simulink model "CSAD_PIDcontroller_ny"  (R2016b)
settings: Solver=ode3  StartTime=0.0  StopTime=tend  FixedStep=0.01  RelTol=1e-3  EnableMultiTasking=on
undefined symbols (not defined in the file): C, Cdn, Cdt, Cmn, d, D, depCur, des_pos, E, emfact, eps_c, epsilon, hd, hd2, Hoerner, I_s, k_cc, K_d_psi, K_d_x, K_d_y, K_i_psi, K_i_x, K_i_y, K_omega, K_p_psi, K_p_x, K_p_y, Kp, Kq, Kqr, Kt, Ktr, L, Max_Acceleration, Max_rotation, Max_thrust, moorLineProp, n_c, n_max, p_cc, P_max, Q_f0, Q_max, r0, r_cc, r_dot0, rBottomEnd, Rho, rhoCab, rhoWat, stiffSeafloor, T_psi, T_x, T_y, Thruster, Thruster_control, Thruster_lock, velCur, vessel, vesselABC ... (+7)
libraries: marine_gnc x9, dspmtrx3 x6, simulink x6, simulink_extras x3, marine_hydro x3
(part 3 of 5)

== matlab function CSAD_PIDcontroller_ny/Virtual CS Inocean Cat I Drillship 6 DOF/FEM mooring/Mooring Line 2/FEM mooring cable ==
  data: state input; rBottomEnd input; rTopEnd input; state_dot output; E input; d input; L input; rhoCab input; rhoWat input; emfact input; stiffSeafloor input; Cmn input; Cdt input; Cdn input; depCur input; velCur input; Ftop output; waterDepth input
function [state_dot, Ftop]  = fcn(state,rBottomEnd,rTopEnd,E,d,L,rhoCab,rhoWat,emfact,stiffSeafloor,Cmn,Cdt,Cdn,depCur,velCur,waterDepth)
% This is a sophisticated FEM model which is used to describe the cable. It
% contain the following parameters.
%   Coordinate
%       local NED reference: calm water sea surface z=0, positive upward

%   Outputs:
%       r_ddot	---     acceleration of each nodes
%       Ftop	---     top end restoring force
%       Fbottom ---     bottom end restoring force

%   Input variables:
%       r       ---     positions of nodes [3*(numNode-1),1]
%       r_dot   ---     velocities of nodes [3*(numNode-1),1]
%       rBottomEnd	--- bottom point       [3,1]
%       topEnd      --- top point       [3,1]

%   Initial conditions:
%       r0      ---     initial positionsof nodes   [3*(numNode),1]
%       r_dot0  ---     initial velocities of nodes [3*(numNode),1]

%   Constant parameters:
%       E       ---     elastic modulus
%       d       ---     diameter of the cable
%       A0      ---     area of the cable (A0=pi/4*d^2)
%       L       ---     length of the cable
%       numNode	---     number of the nodes (excluded the anchor)        
%       rhoCab	---     cable density
%       rhoWat	---     water density
%       ef      ---     factor for stiffness calculation in the reaction force,[1,1], e.g. ef=1;
%       Cmn     ---     added mass coefficient in mass matrix, [1,1]
%       Cdt     ---     tangential drag coefficient in drag force, [1,1]
%       Cdn     ---     normal drag coefficient in drag force, [1,1]
%       depCur  ---     current depth vector (botom to water surface)  [numCur,1]
%       velCur  ---     current velocity vector             [3*numCur,1]
%       deltaT  ---     time difference between two process, [1,1]

%   Other parameters in the program:
%       l       ---     length of each segment, [numNode-1,1]  
%       l_k   --- 	[3*(numNode-1),1]           Eq.9
%       epsilon_k   ---     strain, [numNode-1,1]     Eq.9
%       rho0    ---     mass per unit length of unstrethched cable, [1,1]
%       vc      ---     velicity of current at each node, [3*(numCur+1),1]
%       numCur  ---     number of point in the current profile
%       numNodeSeaFloor     --- number of node on the sea floor
%       f_k_r   ---     reaction force at each node, [3*(numCur+1),1]               Eq.17
%       f_k_hg  ---     hydrostatic force & gravity at each node, [3*(numCur+1),1]  Eq.17
%       f_k_d   ---     drag force at each node, [3*(numCur+1),1]                   Eq.17
%       P_k     ---     (l_k*l_k')/epsilon_k^2                                      Eq.19
%       m_k     ---     mass matrix of each node, [3,3]
%       r_ddot  ---     acceleration of nodes [3*(numNode+1),1]                     Eq.17


%   Note that :
	 % i=k in {l_k,epsilon_k,vc,f_k_r,f_k_hg,f_k_g,r,r_dot,m_k} [k=1,...,n-1],
            
%   Reference:
%       Aamo, O. M. and T. I. Fossen (2001). "Finite Element Modelling of 
%       Moored Vessels." Mathematical and Computer Modelling of Dynamical 
%       Systems 7(1): 47-75.

% Author: Zhengru Ren, NTNU
%% Constants statement
numNode     =   20;
% persistent numNode
% if isempty(numNode)
% numNode=numNode1;
% end

l   =   L/numNode*ones(1,numNode);      % length per segment (m)
g   =   9.81;                           % gravity acceleration (m/s^2)
A0  =   pi/4*d^2;                       % area (m^2)
rho0=   rhoCab*A0; 
C1  =   Cmn*A0*rhoWat;
C2  =   0.5*Cdt*d*rhoWat;
C3  =   0.5*Cdn*d*rhoWat;

r   =   state(1:3*numNode-3);
r_dot   =   state(3*numNode-2:6*numNode-6);

%% Current velocity resample for each node
vc      =   zeros(3*(numNode-1),1);
for i = 1 : numNode-1
    if r(3*i)  >  waterDepth
        vc(3*i-2:3*i)   =  [0;0;0]; % below or on the seafloor
    elseif r(3*i)  >=  depCur(end) % below the bottom current point (below the seabed)
        vc(3*i-2:3*i)   =  velCur(end-2:end);
    elseif  r(3*i)  <=  depCur(1) % above the top current point (above water surface)
        vc(3*i-2:3*i)   =   velCur(1:3);
    else
        cur=max(find(depCur<=r(3*i)));       
        vc(3*i-2:3*i)   =   velCur(3*cur-2:3*cur)+...
            (velCur(3*cur+1:3*cur+3)-velCur(3*cur-2:3*cur))./...
            (depCur(cur+1)-depCur(cur)).*(r(3*i)-depCur(cur));
    end
end
% r(3:3:end)
% vc
%% Basic parameter update
l_k         =   zeros(3*numNode,1);
epsilon_k   =   zeros(numNode,1);

l_k(1:3,1)	=	r(1:3,1)-rBottomEnd;
epsilon_k(1,1)      =   norm(l_k(1:3,1),2);
for i = 2 : numNode-1
    l_k(3*i-2:3*i,1)    =   r(3*i-2:3*i,1)-r(3*(i-1)-2:3*(i-1),1); % [NOTE]
    epsilon_k(i,1)      =   norm(l_k(3*i-2:3*i,1),2);
end
l_k(3*numNode-2:3*numNode,1)	=	rTopEnd-r(3*(numNode-1)-2:3*(numNode-1),1);
epsilon_k(numNode,1)      =   norm(l_k(3*numNode-2:3*numNode,1),2);


%% External forces
% Reaction force
f_k_r       =   zeros(3*(numNode),1);
f_k_hg      =   zeros(3*(numNode),1);
f_k_d       =   zeros(3*(numNode),1);
f_tol       =   zeros(3*(numNode),1);
r_ddot  =   zeros(3*(numNode-1),1);

f_k_hg(3)	=	f_k_hg(3)+0.5*l(1)*A0*(rhoCab-rhoWat)*g;
f_k_r(1:3)	=   f_k_r(1:3)-E*A0*emfact*((1/l(1)-1/epsilon_k(1))*l_k(1:3));
for i = 1:numNode-1
    f_k_r(3*i-2:3*i)	=   f_k_r(3*i-2:3*i)+E*A0*emfact*((1/l(i+1)-1/epsilon_k(i+1))*l_k(3*i+1:3*i+3));
    f_k_r(3*i+1:3*i+3)	=   f_k_r(3*i+1:3*i+3)-E*A0*emfact*((1/l(i+1)-1/epsilon_k(i+1))*l_k(3*i+1:3*i+3));
    %     E*A0*emfact*((1/l(i)-1/epsilon_k(i))*l_k(3*i-2:3*i) - (1/l(i+1)-1/epsilon_k(i+1))*l_k(3*i+1:3*i+3));
    

    % Hydrostatic force & gravity
    if r(3*i) < waterDepth-2  % above the seafloor(-2 safety value)
        f_k_hg(3*i)	=	f_k_hg(3*i)+0.5*l(i+1)*A0*(rhoCab-rhoWat)*g;
        f_k_hg(3*i+3)	=	f_k_hg(3*i+3)+0.5*l(i+1)*A0*(rhoCab-rhoWat)*g;
    else % below or on the seafloor
        f_k_hg(3*i)	=   stiffSeafloor*(waterDepth-r(3*i));
    end

    % Drag force
    P_k         =   l_k(3*i-2:3*i)*l_k(3*i-2:3*i)'./(epsilon_k(i)^2);
    P_kplus1    =   l_k(3*i+1:3*i+3)*l_k(3*i+1:3*i+3)'./(epsilon_k(i+1)^2); 
    f_k_d(3*i-2:3*i)	=   -0.5*(  C2*(...
                                abs((r_dot(3*i-2:3*i)-vc(3*i-2:3*i))'*l_k(3*i-2:3*i))*P_k+...
                                abs((r_dot(3*i-2:3*i)-vc(3*i-2:3*i))'*l_k(3*i+1:3*i+3))*P_kplus1...
                                        )...   % dt
                                 +  C3*(...
                                epsilon_k(i)*norm((eye(3)-P_k)*(r_dot(3*i-2:3*i)-vc(3*i-2:3*i)))*(eye(3)-P_k)+...
                                epsilon_k(i+1)*norm((eye(3)-P_kplus1)*(r_dot(3*i-2:3*i)-vc(3*i-2:3*i)))*(eye(3)-P_kplus1)...
                                        )...    % dn
                                )*(r_dot(3*i-2:3*i)-vc(3*i-2:3*i));
                            
    f_tol(3*i-2:3*i)   =   f_k_hg(3*i-2:3*i)+f_k_d(3*i-2:3*i)+f_k_r(3*i-2:3*i); 	% total force
                        
	m_k     =   (rho0*l(i)+0.5*C1*(epsilon_k(i)+epsilon_k(i+1)))*eye(3)-0.5*C1*(l_k(3*i-2:3*i)*l_k(3*i-2:3*i)'/epsilon_k(i)+l_k(3*i+1:3*i+3)*l_k(3*i+1:3*i+3)'/epsilon_k(i+1));
	AAA=(m_k(3,3)*m_k(1,2)^2 - 2*m_k(1,2)*m_k(1,3)*m_k(2,3) + m_k(2,2)*m_k(1,3)^2 + m_k(1,1)*m_k(2,3)^2 - m_k(1,1)*m_k(2,2)*m_k(3,3));
    r_ddot(3*i-2:3*i,1)	=   [ -(- m_k(2,3)^2 + m_k(2,2)*m_k(3,3))/AAA,    (m_k(1,2)*m_k(3,3) - m_k(1,3)*m_k(2,3))/AAA,   -(m_k(1,2)*m_k(2,3) - m_k(1,3)*m_k(2,2))/AAA;
        (m_k(1,2)*m_k(3,3) - m_k(1,3)*m_k(2,3))/AAA, -(- m_k(1,3)^2 + m_k(1,1)*m_k(3,3))/AAA,   -(m_k(1,2)*m_k(1,3) - m_k(1,1)*m_k(2,3))/AAA;
        -(m_k(1,2)*m_k(2,3) - m_k(1,3)*m_k(2,2))/AAA,   -(m_k(1,2)*m_k(1,3) - m_k(1,1)*m_k(2,3))/AAA, -(- m_k(1,2)^2 + m_k(1,1)*m_k(2,2))/AAA]*f_tol(3*i-2:3*i);
end


%% Mass matrix & acceleration
% for i = 1:numNode-1
%     m_k     =   (rho0*l(i)+0.5*C1*(epsilon_k(i)+epsilon_k(i+1)))*eye(3)-0.5*C1*(l_k(3*i-2:3*i)*l_k(3*i-2:3*i)'/epsilon_k(i)+l_k(3*i+1:3*i+3)*l_k(3*i+1:3*i+3)'/epsilon_k(i+1));
% %   (1)     r_ddot(3*i-2:3*i,1)	=	m_k\f_tol(3*i-2:3*i);
% %   (2)     
% AAA=(m_k(3,3)*m_k(1,2)^2 - 2*m_k(1,2)*m_k(1,3)*m_k(2,3) + m_k(2,2)*m_k(1,3)^2 + m_k(1,1)*m_k(2,3)^2 - m_k(1,1)*m_k(2,2)*m_k(3,3));
% r_ddot(3*i-2:3*i,1)	=   [ -(- m_k(2,3)^2 + m_k(2,2)*m_k(3,3))/AAA,    (m_k(1,2)*m_k(3,3) - m_k(1,3)*m_k(2,3))/AAA,   -(m_k(1,2)*m_k(2,3) - m_k(1,3)*m_k(2,2))/AAA;
%     (m_k(1,2)*m_k(3,3) - m_k(1,3)*m_k(2,3))/AAA, -(- m_k(1,3)^2 + m_k(1,1)*m_k(3,3))/AAA,   -(m_k(1,2)*m_k(1,3) - m_k(1,1)*m_k(2,3))/AAA;
%     -(m_k(1,2)*m_k(2,3) - m_k(1,3)*m_k(2,2))/AAA,   -(m_k(1,2)*m_k(1,3) - m_k(1,1)*m_k(2,3))/AAA, -(- m_k(1,2)^2 + m_k(1,1)*m_k(2,2))/AAA]*f_tol(3*i-2:3*i);
% 
% %   (3)
% % m1=[m_k(1,1),m_k(1,2),m_k(1,3),m_k(2,2),m_k(2,3),m_k(3,3)];F=f_tol(3*i-2:3*i);
% % a12=m_k(1,2);a13=m_k(1,3);a23=m_k(2,3);
% % m1(2)=m1(2)/m1(1);
% % m1(3)=m1(3)/m1(1);
% % F(1)=F(1)/m1(1);
% % m1(5)=(m1(5)-a12*m1(3))/(m1(4)-a12*m1(2));
% % F(2)=(F(2)-a12*F(1))/(m1(4)-a12*m1(2));		
% % m1(6)=m1(6)-a13*m1(3)-m1(5)*(a23-a13*m1(2));
% % r_ddot(3*i,1)=(F(3)-a13*F(1)-F(2)*(a23-a13*m1(2)))/m1(6);
% % r_ddot(3*i-1,1)=F(2)-m1(5)*F(3);
% % r_ddot(3*i-2,1)=F(1)-m1(2)*F(2)+m1(3)*F(3);    
% end

state_dot = [r_dot;r_ddot];

%% Seafloor resample for each node (if the seafloor is not flat)
% numNodeSeaFloor     =
% xNodeSeaFloor	=   zeros(numNodeSeaFloor,1);
% yNodeSeaFloor	=   zeros(numNodeSeaFloor,1);
% zNodeSeaFloorZ	=   zeros(numNodeSeaFloor,1);
% 
% for i=1:numNodeSeaFloor
%     xNodeSeaFloor(i,1)	=	r(3*i-2,1);
%     yNodeSeaFloor(i,1)	=   r(3*i-2,1);
% end
% zNodeSeaFloorZ  =   interp2(seaFloor(:,1),seaFloor(:,2),seaFloor(:,3),xNodeSeaFloor,yNodeSeaFloor);
% zNodeSeaFloorZ   =   waterDepth*ones(numNode+1,1);

%% Restoring forces at the top end and bottom end
% Bottom end
% Fbottom         =   E*A0*emfact*(1/l(1)-1/epsilon_k(1)) * l_k(1:3);

% Top end
Ftop            =   -E*A0*emfact*(1/l(numNode)-1/epsilon_k(numNode)) * l_k(3*numNode-2:3*numNode);

== matlab function CSAD_PIDcontroller_ny/Virtual CS Inocean Cat I Drillship 6 DOF/FEM mooring/Mooring Line 1/FEM mooring cable ==
  data: state input; rBottomEnd input; rTopEnd input; state_dot output; E input; d input; L input; rhoCab input; rhoWat input; emfact input; stiffSeafloor input; Cmn input; Cdt input; Cdn input; depCur input; velCur input; Ftop output; waterDepth input
function [state_dot, Ftop]  = fcn(state,rBottomEnd,rTopEnd,E,d,L,rhoCab,rhoWat,emfact,stiffSeafloor,Cmn,Cdt,Cdn,depCur,velCur,waterDepth)
% This is a sophisticated FEM model which is used to describe the cable. It
% contain the following parameters.
%   Coordinate
%       local NED reference: calm water sea surface z=0, positive upward

%   Outputs:
%       r_ddot	---     acceleration of each nodes
%       Ftop	---     top end restoring force
%       Fbottom ---     bottom end restoring force

%   Input variables:
%       r       ---     positions of nodes [3*(numNode-1),1]
%       r_dot   ---     velocities of nodes [3*(numNode-1),1]
%       rBottomEnd	--- bottom point       [3,1]
%       rtopEnd      --- top point       [3,1]

%   Initial conditions:
%       r0      ---     initial positionsof nodes   [3*(numNode),1]
%       r_dot0  ---     initial velocities of nodes [3*(numNode),1]

%   Constant parameters:
%       E       ---     elastic modulus
%       d       ---     diameter of the cable
%       A0      ---     area of the cable (A0=pi/4*d^2)
%       L       ---     length of the cable
%       numNode	---     number of the nodes (excluded the anchor)        
%       rhoCab	---     cable density
%       rhoWat	---     water density
%       ef      ---     factor for stiffness calculation in the reaction force,[1,1], e.g. ef=1;
%       Cmn     ---     added mass coefficient in mass matrix, [1,1]
%       Cdt     ---     tangential drag coefficient in drag force, [1,1]
%       Cdn     ---     normal drag coefficient in drag force, [1,1]
%       depCur  ---     current depth vector (botom to water surface)  [numCur,1]
%       velCur  ---     current velocity vector             [3*numCur,1]
%       deltaT  ---     time difference between two process, [1,1]

%   Other parameters in the program:
%       l       ---     length of each segment, [numNode-1,1]  
%       l_k   --- 	[3*(numNode-1),1]           Eq.9
%       epsilon_k   ---     strain, [numNode-1,1]     Eq.9
%       rho0    ---     mass per unit length of unstrethched cable, [1,1]
%       vc      ---     velicity of current at each node, [3*(numCur+1),1]
%       numCur  ---     number of point in the current profile
%       numNodeSeaFloor     --- number of node on the sea floor
%       f_k_r   ---     reaction force at each node, [3*(numCur+1),1]               Eq.17
%       f_k_hg  ---     hydrostatic force & gravity at each node, [3*(numCur+1),1]  Eq.17
%       f_k_d   ---     drag force at each node, [3*(numCur+1),1]                   Eq.17
%       P_k     ---     (l_k*l_k')/epsilon_k^2                                      Eq.19
%       m_k     ---     mass matrix of each node, [3,3]
%       r_ddot  ---     acceleration of nodes [3*(numNode+1),1]                     Eq.17


%   Note that :
	 % i=k in {l_k,epsilon_k,vc,f_k_r,f_k_hg,f_k_g,r,r_dot,m_k} [k=1,...,n-1],
            
%   Reference:
%       Aamo, O. M. and T. I. Fossen (2001). "Finite Element Modelling of 
%       Moored Vessels." Mathematical and Computer Modelling of Dynamical 
%       Systems 7(1): 47-75.

% Author: Zhengru Ren, NTNU
%% Constants statement
numNode     =   20;
% persistent numNode
% if isempty(numNode)
% numNode=numNode1;
% end

l   =   L/numNode*ones(1,numNode);      % length per segment (m)
g   =   9.81;                           % gravity acceleration (m/s^2)
A0  =   pi/4*d^2;                       % area (m^2)
rho0=   rhoCab*A0; 
C1  =   Cmn*A0*rhoWat;
C2  =   0.5*Cdt*d*rhoWat;
C3  =   0.5*Cdn*d*rhoWat;

r   =   state(1:3*numNode-3);
r_dot   =   state(3*numNode-2:6*numNode-6);

%% Current velocity resample for each node
vc      =   zeros(3*(numNode-1),1);
for i = 1 : numNode-1
    if r(3*i)  >  waterDepth
        vc(3*i-2:3*i)   =  [0;0;0]; % below or on the seafloor
    elseif r(3*i)  >=  depCur(end) % below the bottom current point (below the seabed)
        vc(3*i-2:3*i)   =  velCur(end-2:end);
    elseif  r(3*i)  <=  depCur(1) % above the top current point (above water surface)
        vc(3*i-2:3*i)   =   velCur(1:3);
    else
        cur=max(find(depCur<=r(3*i)));       
        vc(3*i-2:3*i)   =   velCur(3*cur-2:3*cur)+...
            (velCur(3*cur+1:3*cur+3)-velCur(3*cur-2:3*cur))./...
            (depCur(cur+1)-depCur(cur)).*(r(3*i)-depCur(cur));
    end
end
% r(3:3:end)
% vc
%% Basic parameter update
l_k         =   zeros(3*numNode,1);
epsilon_k   =   zeros(numNode,1);

l_k(1:3,1)	=	r(1:3,1)-rBottomEnd;
epsilon_k(1,1)      =   norm(l_k(1:3,1),2);
for i = 2 : numNode-1
    l_k(3*i-2:3*i,1)    =   r(3*i-2:3*i,1)-r(3*(i-1)-2:3*(i-1),1); % [NOTE]
    epsilon_k(i,1)      =   norm(l_k(3*i-2:3*i,1),2);
end
l_k(3*numNode-2:3*numNode,1)	=	rTopEnd-r(3*(numNode-1)-2:3*(numNode-1),1);
epsilon_k(numNode,1)      =   norm(l_k(3*numNode-2:3*numNode,1),2);


%% External forces
% Reaction force
f_k_r       =   zeros(3*(numNode),1);
f_k_hg      =   zeros(3*(numNode),1);
f_k_d       =   zeros(3*(numNode),1);
f_tol       =   zeros(3*(numNode),1);
r_ddot      =   zeros(3*(numNode-1),1);

f_k_hg(3)	=	f_k_hg(3)+0.5*l(1)*A0*(rhoCab-rhoWat)*g;
f_k_r(1:3)	=   f_k_r(1:3)-E*A0*emfact*((1/l(1)-1/epsilon_k(1))*l_k(1:3));
for i = 1:numNode-1
    f_k_r(3*i-2:3*i)	=   f_k_r(3*i-2:3*i)+E*A0*emfact*((1/l(i+1)-1/epsilon_k(i+1))*l_k(3*i+1:3*i+3));
    f_k_r(3*i+1:3*i+3)	=   f_k_r(3*i+1:3*i+3)-E*A0*emfact*((1/l(i+1)-1/epsilon_k(i+1))*l_k(3*i+1:3*i+3));
    %     E*A0*emfact*((1/l(i)-1/epsilon_k(i))*l_k(3*i-2:3*i) - (1/l(i+1)-1/epsilon_k(i+1))*l_k(3*i+1:3*i+3));
    

    % Hydrostatic force & gravity
    if r(3*i) < waterDepth-2  % above the seafloor(-2 safety value)
        f_k_hg(3*i)	=	f_k_hg(3*i)+0.5*l(i+1)*A0*(rhoCab-rhoWat)*g;
        f_k_hg(3*i+3)	=	f_k_hg(3*i+3)+0.5*l(i+1)*A0*(rhoCab-rhoWat)*g;
    else % below or on the seafloor
        f_k_hg(3*i)	=   stiffSeafloor*(waterDepth-r(3*i));
    end

    % Drag force
    P_k         =   l_k(3*i-2:3*i)*l_k(3*i-2:3*i)'./(epsilon_k(i)^2);
    P_kplus1    =   l_k(3*i+1:3*i+3)*l_k(3*i+1:3*i+3)'./(epsilon_k(i+1)^2); 
    f_k_d(3*i-2:3*i)	=   -0.5*(  C2*(...
                                abs((r_dot(3*i-2:3*i)-vc(3*i-2:3*i))'*l_k(3*i-2:3*i))*P_k+...
                                abs((r_dot(3*i-2:3*i)-vc(3*i-2:3*i))'*l_k(3*i+1:3*i+3))*P_kplus1...
                                        )...   % dt
                                 +  C3*(...
                                epsilon_k(i)*norm((eye(3)-P_k)*(r_dot(3*i-2:3*i)-vc(3*i-2:3*i)))*(eye(3)-P_k)+...
                                epsilon_k(i+1)*norm((eye(3)-P_kplus1)*(r_dot(3*i-2:3*i)-vc(3*i-2:3*i)))*(eye(3)-P_kplus1)...
                                        )...    % dn
                                )*(r_dot(3*i-2:3*i)-vc(3*i-2:3*i));
                            
    f_tol(3*i-2:3*i)   =   f_k_hg(3*i-2:3*i)+f_k_d(3*i-2:3*i)+f_k_r(3*i-2:3*i); 	% total force
                        
	m_k     =   (rho0*l(i)+0.5*C1*(epsilon_k(i)+epsilon_k(i+1)))*eye(3)-0.5*C1*(l_k(3*i-2:3*i)*l_k(3*i-2:3*i)'/epsilon_k(i)+l_k(3*i+1:3*i+3)*l_k(3*i+1:3*i+3)'/epsilon_k(i+1));
	AAA=(m_k(3,3)*m_k(1,2)^2 - 2*m_k(1,2)*m_k(1,3)*m_k(2,3) + m_k(2,2)*m_k(1,3)^2 + m_k(1,1)*m_k(2,3)^2 - m_k(1,1)*m_k(2,2)*m_k(3,3));
    r_ddot(3*i-2:3*i,1)	=   [ -(- m_k(2,3)^2 + m_k(2,2)*m_k(3,3))/AAA,    (m_k(1,2)*m_k(3,3) - m_k(1,3)*m_k(2,3))/AAA,   -(m_k(1,2)*m_k(2,3) - m_k(1,3)*m_k(2,2))/AAA;
        (m_k(1,2)*m_k(3,3) - m_k(1,3)*m_k(2,3))/AAA, -(- m_k(1,3)^2 + m_k(1,1)*m_k(3,3))/AAA,   -(m_k(1,2)*m_k(1,3) - m_k(1,1)*m_k(2,3))/AAA;
        -(m_k(1,2)*m_k(2,3) - m_k(1,3)*m_k(2,2))/AAA,   -(m_k(1,2)*m_k(1,3) - m_k(1,1)*m_k(2,3))/AAA, -(- m_k(1,2)^2 + m_k(1,1)*m_k(2,2))/AAA]*f_tol(3*i-2:3*i);
end


%% Mass matrix & acceleration
% for i = 1:numNode-1
%     m_k     =   (rho0*l(i)+0.5*C1*(epsilon_k(i)+epsilon_k(i+1)))*eye(3)-0.5*C1*(l_k(3*i-2:3*i)*l_k(3*i-2:3*i)'/epsilon_k(i)+l_k(3*i+1:3*i+3)*l_k(3*i+1:3*i+3)'/epsilon_k(i+1));
% %   (1)     r_ddot(3*i-2:3*i,1)	=	m_k\f_tol(3*i-2:3*i);
% %   (2)     
% AAA=(m_k(3,3)*m_k(1,2)^2 - 2*m_k(1,2)*m_k(1,3)*m_k(2,3) + m_k(2,2)*m_k(1,3)^2 + m_k(1,1)*m_k(2,3)^2 - m_k(1,1)*m_k(2,2)*m_k(3,3));
% r_ddot(3*i-2:3*i,1)	=   [ -(- m_k(2,3)^2 + m_k(2,2)*m_k(3,3))/AAA,    (m_k(1,2)*m_k(3,3) - m_k(1,3)*m_k(2,3))/AAA,   -(m_k(1,2)*m_k(2,3) - m_k(1,3)*m_k(2,2))/AAA;
%     (m_k(1,2)*m_k(3,3) - m_k(1,3)*m_k(2,3))/AAA, -(- m_k(1,3)^2 + m_k(1,1)*m_k(3,3))/AAA,   -(m_k(1,2)*m_k(1,3) - m_k(1,1)*m_k(2,3))/AAA;
%     -(m_k(1,2)*m_k(2,3) - m_k(1,3)*m_k(2,2))/AAA,   -(m_k(1,2)*m_k(1,3) - m_k(1,1)*m_k(2,3))/AAA, -(- m_k(1,2)^2 + m_k(1,1)*m_k(2,2))/AAA]*f_tol(3*i-2:3*i);
% 
% %   (3)
% % m1=[m_k(1,1),m_k(1,2),m_k(1,3),m_k(2,2),m_k(2,3),m_k(3,3)];F=f_tol(3*i-2:3*i);
% % a12=m_k(1,2);a13=m_k(1,3);a23=m_k(2,3);
% % m1(2)=m1(2)/m1(1);
% % m1(3)=m1(3)/m1(1);
% % F(1)=F(1)/m1(1);
% % m1(5)=(m1(5)-a12*m1(3))/(m1(4)-a12*m1(2));
% % F(2)=(F(2)-a12*F(1))/(m1(4)-a12*m1(2));		
% % m1(6)=m1(6)-a13*m1(3)-m1(5)*(a23-a13*m1(2));
% % r_ddot(3*i,1)=(F(3)-a13*F(1)-F(2)*(a23-a13*m1(2)))/m1(6);
% % r_ddot(3*i-1,1)=F(2)-m1(5)*F(3);
% % r_ddot(3*i-2,1)=F(1)-m1(2)*F(2)+m1(3)*F(3);    
% end

state_dot = [r_dot;r_ddot];

%% Seafloor resample for each node (if the seafloor is not flat)
% numNodeSeaFloor     =
% xNodeSeaFloor	=   zeros(numNodeSeaFloor,1);
% yNodeSeaFloor	=   zeros(numNodeSeaFloor,1);
% zNodeSeaFloorZ	=   zeros(numNodeSeaFloor,1);
% 
% for i=1:numNodeSeaFloor
%     xNodeSeaFloor(i,1)	=	r(3*i-2,1);
%     yNodeSeaFloor(i,1)	=   r(3*i-2,1);
% end
% zNodeSeaFloorZ  =   interp2(seaFloor(:,1),seaFloor(:,2),seaFloor(:,3),xNodeSeaFloor,yNodeSeaFloor);
% zNodeSeaFloorZ   =   waterDepth*ones(numNode+1,1);

%% Restoring forces at the top end and bottom end
% Bottom end
% Fbottom         =   E*A0*emfact*(1/l(1)-1/epsilon_k(1)) * l_k(1:3);

% Top end
Ftop            =   -E*A0*emfact*(1/l(numNode)-1/epsilon_k(numNode)) * l_k(3*numNode-2:3*numNode);

== matlab function CSAD_PIDcontroller_ny/Virtual CS Inocean Cat I Drillship 6 DOF/FEM mooring/Mooring Line 3/FEM mooring cable ==
  data: state input; rBottomEnd input; rTopEnd input; state_dot output; E input; d input; L input; rhoCab input; rhoWat input; emfact input; stiffSeafloor input; Cmn input; Cdt input; Cdn input; depCur input; velCur input; Ftop output; waterDepth input
function [state_dot, Ftop]  = fcn(state,rBottomEnd,rTopEnd,E,d,L,rhoCab,rhoWat,emfact,stiffSeafloor,Cmn,Cdt,Cdn,depCur,velCur,waterDepth)
% This is a sophisticated FEM model which is used to describe the cable. It
% contain the following parameters.
%   Coordinate
%       local NED reference: calm water sea surface z=0, positive upward

%   Outputs:
%       r_ddot	---     acceleration of each nodes
%       Ftop	---     top end restoring force
%       Fbottom ---     bottom end restoring force

%   Input variables:
%       r       ---     positions of nodes [3*(numNode-1),1]
%       r_dot   ---     velocities of nodes [3*(numNode-1),1]
%       rBottomEnd	--- bottom point       [3,1]
%       topEnd      --- top point       [3,1]

%   Initial conditions:
%       r0      ---     initial positionsof nodes   [3*(numNode),1]
%       r_dot0  ---     initial velocities of nodes [3*(numNode),1]

%   Constant parameters:
%       E       ---     elastic modulus
%       d       ---     diameter of the cable
%       A0      ---     area of the cable (A0=pi/4*d^2)
%       L       ---     length of the cable
%       numNode	---     number of the nodes (excluded the anchor)        
%       rhoCab	---     cable density
%       rhoWat	---     water density
%       ef      ---     factor for stiffness calculation in the reaction force,[1,1], e.g. ef=1;
%       Cmn     ---     added mass coefficient in mass matrix, [1,1]
%       Cdt     ---     tangential drag coefficient in drag force, [1,1]
%       Cdn     ---     normal drag coefficient in drag force, [1,1]
%       depCur  ---     current depth vector (botom to water surface)  [numCur,1]
%       velCur  ---     current velocity vector             [3*numCur,1]
%       deltaT  ---     time difference between two process, [1,1]

%   Other parameters in the program:
%       l       ---     length of each segment, [numNode-1,1]  
%       l_k   --- 	[3*(numNode-1),1]           Eq.9
%       epsilon_k   ---     strain, [numNode-1,1]     Eq.9
%       rho0    ---     mass per unit length of unstrethched cable, [1,1]
%       vc      ---     velicity of current at each node, [3*(numCur+1),1]
%       numCur  ---     number of point in the current profile
%       numNodeSeaFloor     --- number of node on the sea floor
%       f_k_r   ---     reaction force at each node, [3*(numCur+1),1]               Eq.17
%       f_k_hg  ---     hydrostatic force & gravity at each node, [3*(numCur+1),1]  Eq.17
%       f_k_d   ---     drag force at each node, [3*(numCur+1),1]                   Eq.17
%       P_k     ---     (l_k*l_k')/epsilon_k^2                                      Eq.19
%       m_k     ---     mass matrix of each node, [3,3]
%       r_ddot  ---     acceleration of nodes [3*(numNode+1),1]                     Eq.17


%   Note that :
	 % i=k in {l_k,epsilon_k,vc,f_k_r,f_k_hg,f_k_g,r,r_dot,m_k} [k=1,...,n-1],
            
%   Reference:
%       Aamo, O. M. and T. I. Fossen (2001). "Finite Element Modelling of 
%       Moored Vessels." Mathematical and Computer Modelling of Dynamical 
%       Systems 7(1): 47-75.

% Author: Zhengru Ren, NTNU
%% Constants statement
numNode     =   20;
% persistent numNode
% if isempty(numNode)
% numNode=numNode1;
% end

l   =   L/numNode*ones(1,numNode);      % length per segment (m)
g   =   9.81;                           % gravity acceleration (m/s^2)
A0  =   pi/4*d^2;                       % area (m^2)
rho0=   rhoCab*A0; 
C1  =   Cmn*A0*rhoWat;
C2  =   0.5*Cdt*d*rhoWat;
C3  =   0.5*Cdn*d*rhoWat;

r   =   state(1:3*numNode-3);
r_dot   =   state(3*numNode-2:6*numNode-6);

%% Current velocity resample for each node
vc      =   zeros(3*(numNode-1),1);
for i = 1 : numNode-1
    if r(3*i)  >  waterDepth
        vc(3*i-2:3*i)   =  [0;0;0]; % below or on the seafloor
    elseif r(3*i)  >=  depCur(end) % below the bottom current point (below the seabed)
        vc(3*i-2:3*i)   =  velCur(end-2:end);
    elseif  r(3*i)  <=  depCur(1) % above the top current point (above water surface)
        vc(3*i-2:3*i)   =   velCur(1:3);
    else
        cur=max(find(depCur<=r(3*i)));       
        vc(3*i-2:3*i)   =   velCur(3*cur-2:3*cur)+...
            (velCur(3*cur+1:3*cur+3)-velCur(3*cur-2:3*cur))./...
            (depCur(cur+1)-depCur(cur)).*(r(3*i)-depCur(cur));
    end
end
% r(3:3:end)
% vc
%% Basic parameter update
l_k         =   zeros(3*numNode,1);
epsilon_k   =   zeros(numNode,1);

l_k(1:3,1)	=	r(1:3,1)-rBottomEnd;
epsilon_k(1,1)      =   norm(l_k(1:3,1),2);
for i = 2 : numNode-1
    l_k(3*i-2:3*i,1)    =   r(3*i-2:3*i,1)-r(3*(i-1)-2:3*(i-1),1); % [NOTE]
    epsilon_k(i,1)      =   norm(l_k(3*i-2:3*i,1),2);
end
l_k(3*numNode-2:3*numNode,1)	=	rTopEnd-r(3*(numNode-1)-2:3*(numNode-1),1);
epsilon_k(numNode,1)      =   norm(l_k(3*numNode-2:3*numNode,1),2);


%% External forces
% Reaction force
f_k_r       =   zeros(3*(numNode),1);
f_k_hg      =   zeros(3*(numNode),1);
f_k_d       =   zeros(3*(numNode),1);
f_tol       =   zeros(3*(numNode),1);
r_ddot  =   zeros(3*(numNode-1),1);

f_k_hg(3)	=	f_k_hg(3)+0.5*l(1)*A0*(rhoCab-rhoWat)*g;
f_k_r(1:3)	=   f_k_r(1:3)-E*A0*emfact*((1/l(1)-1/epsilon_k(1))*l_k(1:3));
for i = 1:numNode-1
    f_k_r(3*i-2:3*i)	=   f_k_r(3*i-2:3*i)+E*A0*emfact*((1/l(i+1)-1/epsilon_k(i+1))*l_k(3*i+1:3*i+3));
    f_k_r(3*i+1:3*i+3)	=   f_k_r(3*i+1:3*i+3)-E*A0*emfact*((1/l(i+1)-1/epsilon_k(i+1))*l_k(3*i+1:3*i+3));
    %     E*A0*emfact*((1/l(i)-1/epsilon_k(i))*l_k(3*i-2:3*i) - (1/l(i+1)-1/epsilon_k(i+1))*l_k(3*i+1:3*i+3));
    

    % Hydrostatic force & gravity
    if r(3*i) < waterDepth-2  % above the seafloor(-2 safety value)
        f_k_hg(3*i)	=	f_k_hg(3*i)+0.5*l(i+1)*A0*(rhoCab-rhoWat)*g;
        f_k_hg(3*i+3)	=	f_k_hg(3*i+3)+0.5*l(i+1)*A0*(rhoCab-rhoWat)*g;
    else % below or on the seafloor
        f_k_hg(3*i)	=   stiffSeafloor*(waterDepth-r(3*i));
    end

    % Drag force
    P_k         =   l_k(3*i-2:3*i)*l_k(3*i-2:3*i)'./(epsilon_k(i)^2);
    P_kplus1    =   l_k(3*i+1:3*i+3)*l_k(3*i+1:3*i+3)'./(epsilon_k(i+1)^2); 
    f_k_d(3*i-2:3*i)	=   -0.5*(  C2*(...
                                abs((r_dot(3*i-2:3*i)-vc(3*i-2:3*i))'*l_k(3*i-2:3*i))*P_k+...
                                abs((r_dot(3*i-2:3*i)-vc(3*i-2:3*i))'*l_k(3*i+1:3*i+3))*P_kplus1...
                                        )...   % dt
                                 +  C3*(...
                                epsilon_k(i)*norm((eye(3)-P_k)*(r_dot(3*i-2:3*i)-vc(3*i-2:3*i)))*(eye(3)-P_k)+...
                                epsilon_k(i+1)*norm((eye(3)-P_kplus1)*(r_dot(3*i-2:3*i)-vc(3*i-2:3*i)))*(eye(3)-P_kplus1)...
                                        )...    % dn
                                )*(r_dot(3*i-2:3*i)-vc(3*i-2:3*i));
                            
    f_tol(3*i-2:3*i)   =   f_k_hg(3*i-2:3*i)+f_k_d(3*i-2:3*i)+f_k_r(3*i-2:3*i); 	% total force
                        
	m_k     =   (rho0*l(i)+0.5*C1*(epsilon_k(i)+epsilon_k(i+1)))*eye(3)-0.5*C1*(l_k(3*i-2:3*i)*l_k(3*i-2:3*i)'/epsilon_k(i)+l_k(3*i+1:3*i+3)*l_k(3*i+1:3*i+3)'/epsilon_k(i+1));
	AAA=(m_k(3,3)*m_k(1,2)^2 - 2*m_k(1,2)*m_k(1,3)*m_k(2,3) + m_k(2,2)*m_k(1,3)^2 + m_k(1,1)*m_k(2,3)^2 - m_k(1,1)*m_k(2,2)*m_k(3,3));
    r_ddot(3*i-2:3*i,1)	=   [ -(- m_k(2,3)^2 + m_k(2,2)*m_k(3,3))/AAA,    (m_k(1,2)*m_k(3,3) - m_k(1,3)*m_k(2,3))/AAA,   -(m_k(1,2)*m_k(2,3) - m_k(1,3)*m_k(2,2))/AAA;
        (m_k(1,2)*m_k(3,3) - m_k(1,3)*m_k(2,3))/AAA, -(- m_k(1,3)^2 + m_k(1,1)*m_k(3,3))/AAA,   -(m_k(1,2)*m_k(1,3) - m_k(1,1)*m_k(2,3))/AAA;
        -(m_k(1,2)*m_k(2,3) - m_k(1,3)*m_k(2,2))/AAA,   -(m_k(1,2)*m_k(1,3) - m_k(1,1)*m_k(2,3))/AAA, -(- m_k(1,2)^2 + m_k(1,1)*m_k(2,2))/AAA]*f_tol(3*i-2:3*i);
end


%% Mass matrix & acceleration
% for i = 1:numNode-1
%     m_k     =   (rho0*l(i)+0.5*C1*(epsilon_k(i)+epsilon_k(i+1)))*eye(3)-0.5*C1*(l_k(3*i-2:3*i)*l_k(3*i-2:3*i)'/epsilon_k(i)+l_k(3*i+1:3*i+3)*l_k(3*i+1:3*i+3)'/epsilon_k(i+1));
% %   (1)     r_ddot(3*i-2:3*i,1)	=	m_k\f_tol(3*i-2:3*i);
% %   (2)     
% AAA=(m_k(3,3)*m_k(1,2)^2 - 2*m_k(1,2)*m_k(1,3)*m_k(2,3) + m_k(2,2)*m_k(1,3)^2 + m_k(1,1)*m_k(2,3)^2 - m_k(1,1)*m_k(2,2)*m_k(3,3));
% r_ddot(3*i-2:3*i,1)	=   [ -(- m_k(2,3)^2 + m_k(2,2)*m_k(3,3))/AAA,    (m_k(1,2)*m_k(3,3) - m_k(1,3)*m_k(2,3))/AAA,   -(m_k(1,2)*m_k(2,3) - m_k(1,3)*m_k(2,2))/AAA;
%     (m_k(1,2)*m_k(3,3) - m_k(1,3)*m_k(2,3))/AAA, -(- m_k(1,3)^2 + m_k(1,1)*m_k(3,3))/AAA,   -(m_k(1,2)*m_k(1,3) - m_k(1,1)*m_k(2,3))/AAA;
%     -(m_k(1,2)*m_k(2,3) - m_k(1,3)*m_k(2,2))/AAA,   -(m_k(1,2)*m_k(1,3) - m_k(1,1)*m_k(2,3))/AAA, -(- m_k(1,2)^2 + m_k(1,1)*m_k(2,2))/AAA]*f_tol(3*i-2:3*i);
% 
% %   (3)
% % m1=[m_k(1,1),m_k(1,2),m_k(1,3),m_k(2,2),m_k(2,3),m_k(3,3)];F=f_tol(3*i-2:3*i);
% % a12=m_k(1,2);a13=m_k(1,3);a23=m_k(2,3);
% % m1(2)=m1(2)/m1(1);
% % m1(3)=m1(3)/m1(1);
% % F(1)=F(1)/m1(1);
% % m1(5)=(m1(5)-a12*m1(3))/(m1(4)-a12*m1(2));
% % F(2)=(F(2)-a12*F(1))/(m1(4)-a12*m1(2));		
% % m1(6)=m1(6)-a13*m1(3)-m1(5)*(a23-a13*m1(2));
% % r_ddot(3*i,1)=(F(3)-a13*F(1)-F(2)*(a23-a13*m1(2)))/m1(6);
% % r_ddot(3*i-1,1)=F(2)-m1(5)*F(3);
% % r_ddot(3*i-2,1)=F(1)-m1(2)*F(2)+m1(3)*F(3);    
% end

state_dot = [r_dot;r_ddot];

%% Seafloor resample for each node (if the seafloor is not flat)
% numNodeSeaFloor     =
% xNodeSeaFloor	=   zeros(numNodeSeaFloor,1);
% yNodeSeaFloor	=   zeros(numNodeSeaFloor,1);
% zNodeSeaFloorZ	=   zeros(numNodeSeaFloor,1);
% 
% for i=1:numNodeSeaFloor
%     xNodeSeaFloor(i,1)	=	r(3*i-2,1);
%     yNodeSeaFloor(i,1)	=   r(3*i-2,1);
% end
% zNodeSeaFloorZ  =   interp2(seaFloor(:,1),seaFloor(:,2),seaFloor(:,3),xNodeSeaFloor,yNodeSeaFloor);
% zNodeSeaFloorZ   =   waterDepth*ones(numNode+1,1);

%% Restoring forces at the top end and bottom end
% Bottom end
% Fbottom         =   E*A0*emfact*(1/l(1)-1/epsilon_k(1)) * l_k(1:3);

% Top end
Ftop            =   -E*A0*emfact*(1/l(numNode)-1/epsilon_k(numNode)) * l_k(3*numNode-2:3*numNode);

== matlab function CSAD_PIDcontroller_ny/Virtual CS Inocean Cat I Drillship 6 DOF/FEM mooring/Mooring Line 4/FEM mooring cable ==
  data: state input; rBottomEnd input; rTopEnd input; state_dot output; E input; d input; L input; rhoCab input; rhoWat input; emfact input; stiffSeafloor input; Cmn input; Cdt input; Cdn input; depCur input; velCur input; Ftop output; waterDepth input
function [state_dot, Ftop]  = fcn(state,rBottomEnd,rTopEnd,E,d,L,rhoCab,rhoWat,emfact,stiffSeafloor,Cmn,Cdt,Cdn,depCur,velCur,waterDepth)
% This is a sophisticated FEM model which is used to describe the cable. It
% contain the following parameters.
%   Coordinate
%       local NED reference: calm water sea surface z=0, positive upward

%   Outputs:
%       r_ddot	---     acceleration of each nodes
%       Ftop	---     top end restoring force
%       Fbottom ---     bottom end restoring force

%   Input variables:
%       r       ---     positions of nodes [3*(numNode-1),1]
%       r_dot   ---     velocities of nodes [3*(numNode-1),1]
%       rBottomEnd	--- bottom point       [3,1]
%       topEnd      --- top point       [3,1]

%   Initial conditions:
%       r0      ---     initial positionsof nodes   [3*(numNode),1]
%       r_dot0  ---     initial velocities of nodes [3*(numNode),1]

%   Constant parameters:
%       E       ---     elastic modulus
%       d       ---     diameter of the cable
%       A0      ---     area of the cable (A0=pi/4*d^2)
%       L       ---     length of the cable
%       numNode	---     number of the nodes (excluded the anchor)        
%       rhoCab	---     cable density
%       rhoWat	---     water density
%       ef      ---     factor for stiffness calculation in the reaction force,[1,1], e.g. ef=1;
%       Cmn     ---     added mass coefficient in mass matrix, [1,1]
%       Cdt     ---     tangential drag coefficient in drag force, [1,1]
%       Cdn     ---     normal drag coefficient in drag force, [1,1]
%       depCur  ---     current depth vector (botom to water surface)  [numCur,1]
%       velCur  ---     current velocity vector             [3*numCur,1]
%       deltaT  ---     time difference between two process, [1,1]

%   Other parameters in the program:
%       l       ---     length of each segment, [numNode-1,1]  
%       l_k   --- 	[3*(numNode-1),1]           Eq.9
%       epsilon_k   ---     strain, [numNode-1,1]     Eq.9
%       rho0    ---     mass per unit length of unstrethched cable, [1,1]
%       vc      ---     velicity of current at each node, [3*(numCur+1),1]
%       numCur  ---     number of point in the current profile
%       numNodeSeaFloor     --- number of node on the sea floor
%       f_k_r   ---     reaction force at each node, [3*(numCur+1),1]               Eq.17
%       f_k_hg  ---     hydrostatic force & gravity at each node, [3*(numCur+1),1]  Eq.17
%       f_k_d   ---     drag force at each node, [3*(numCur+1),1]                   Eq.17
%       P_k     ---     (l_k*l_k')/epsilon_k^2                                      Eq.19
%       m_k     ---     mass matrix of each node, [3,3]
%       r_ddot  ---     acceleration of nodes [3*(numNode+1),1]                     Eq.17


%   Note that :
	 % i=k in {l_k,epsilon_k,vc,f_k_r,f_k_hg,f_k_g,r,r_dot,m_k} [k=1,...,n-1],
            
%   Reference:
%       Aamo, O. M. and T. I. Fossen (2001). "Finite Element Modelling of 
%       Moored Vessels." Mathematical and Computer Modelling of Dynamical 
%       Systems 7(1): 47-75.

% Author: Zhengru Ren, NTNU
%% Constants statement
numNode     =   20;
% persistent numNode
% if isempty(numNode)
% numNode=numNode1;
% end

l   =   L/numNode*ones(1,numNode);      % length per segment (m)
g   =   9.81;                           % gravity acceleration (m/s^2)
A0  =   pi/4*d^2;                       % area (m^2)
rho0=   rhoCab*A0; 
C1  =   Cmn*A0*rhoWat;
C2  =   0.5*Cdt*d*rhoWat;
C3  =   0.5*Cdn*d*rhoWat;

r   =   state(1:3*numNode-3);
r_dot   =   state(3*numNode-2:6*numNode-6);

%% Current velocity resample for each node
vc      =   zeros(3*(numNode-1),1);
for i = 1 : numNode-1
    if r(3*i)  >  waterDepth
        vc(3*i-2:3*i)   =  [0;0;0]; % below or on the seafloor
    elseif r(3*i)  >=  depCur(end) % below the bottom current point (below the seabed)
        vc(3*i-2:3*i)   =  velCur(end-2:end);
    elseif  r(3*i)  <=  depCur(1) % above the top current point (above water surface)
        vc(3*i-2:3*i)   =   velCur(1:3);
    else
        cur=max(find(depCur<=r(3*i)));       
        vc(3*i-2:3*i)   =   velCur(3*cur-2:3*cur)+...
            (velCur(3*cur+1:3*cur+3)-velCur(3*cur-2:3*cur))./...
            (depCur(cur+1)-depCur(cur)).*(r(3*i)-depCur(cur));
    end
end
% r(3:3:end)
% vc
%% Basic parameter update
l_k         =   zeros(3*numNode,1);
epsilon_k   =   zeros(numNode,1);

l_k(1:3,1)	=	r(1:3,1)-rBottomEnd;
epsilon_k(1,1)      =   norm(l_k(1:3,1),2);
for i = 2 : numNode-1
    l_k(3*i-2:3*i,1)    =   r(3*i-2:3*i,1)-r(3*(i-1)-2:3*(i-1),1); % [NOTE]
    epsilon_k(i,1)      =   norm(l_k(3*i-2:3*i,1),2);
end
l_k(3*numNode-2:3*numNode,1)	=	rTopEnd-r(3*(numNode-1)-2:3*(numNode-1),1);
epsilon_k(numNode,1)      =   norm(l_k(3*numNode-2:3*numNode,1),2);


%% External forces
% Reaction force
f_k_r       =   zeros(3*(numNode),1);
f_k_hg      =   zeros(3*(numNode),1);
f_k_d       =   zeros(3*(numNode),1);
f_tol       =   zeros(3*(numNode),1);
r_ddot  =   zeros(3*(numNode-1),1);

f_k_hg(3)	=	f_k_hg(3)+0.5*l(1)*A0*(rhoCab-rhoWat)*g;
f_k_r(1:3)	=   f_k_r(1:3)-E*A0*emfact*((1/l(1)-1/epsilon_k(1))*l_k(1:3));
for i = 1:numNode-1
    f_k_r(3*i-2:3*i)	=   f_k_r(3*i-2:3*i)+E*A0*emfact*((1/l(i+1)-1/epsilon_k(i+1))*l_k(3*i+1:3*i+3));
    f_k_r(3*i+1:3*i+3)	=   f_k_r(3*i+1:3*i+3)-E*A0*emfact*((1/l(i+1)-1/epsilon_k(i+1))*l_k(3*i+1:3*i+3));
    %     E*A0*emfact*((1/l(i)-1/epsilon_k(i))*l_k(3*i-2:3*i) - (1/l(i+1)-1/epsilon_k(i+1))*l_k(3*i+1:3*i+3));
    

    % Hydrostatic force & gravity
    if r(3*i) < waterDepth-2  % above the seafloor(-2 safety value)
        f_k_hg(3*i)	=	f_k_hg(3*i)+0.5*l(i+1)*A0*(rhoCab-rhoWat)*g;
        f_k_hg(3*i+3)	=	f_k_hg(3*i+3)+0.5*l(i+1)*A0*(rhoCab-rhoWat)*g;
    else % below or on the seafloor
        f_k_hg(3*i)	=   stiffSeafloor*(waterDepth-r(3*i));
    end

    % Drag force
    P_k         =   l_k(3*i-2:3*i)*l_k(3*i-2:3*i)'./(epsilon_k(i)^2);
    P_kplus1    =   l_k(3*i+1:3*i+3)*l_k(3*i+1:3*i+3)'./(epsilon_k(i+1)^2); 
    f_k_d(3*i-2:3*i)	=   -0.5*(  C2*(...
                                abs((r_dot(3*i-2:3*i)-vc(3*i-2:3*i))'*l_k(3*i-2:3*i))*P_k+...
                                abs((r_dot(3*i-2:3*i)-vc(3*i-2:3*i))'*l_k(3*i+1:3*i+3))*P_kplus1...
                                        )...   % dt
                                 +  C3*(...
                                epsilon_k(i)*norm((eye(3)-P_k)*(r_dot(3*i-2:3*i)-vc(3*i-2:3*i)))*(eye(3)-P_k)+...
                                epsilon_k(i+1)*norm((eye(3)-P_kplus1)*(r_dot(3*i-2:3*i)-vc(3*i-2:3*i)))*(eye(3)-P_kplus1)...
                                        )...    % dn
                                )*(r_dot(3*i-2:3*i)-vc(3*i-2:3*i));
                            
    f_tol(3*i-2:3*i)   =   f_k_hg(3*i-2:3*i)+f_k_d(3*i-2:3*i)+f_k_r(3*i-2:3*i); 	% total force
                        
	m_k     =   (rho0*l(i)+0.5*C1*(epsilon_k(i)+epsilon_k(i+1)))*eye(3)-0.5*C1*(l_k(3*i-2:3*i)*l_k(3*i-2:3*i)'/epsilon_k(i)+l_k(3*i+1:3*i+3)*l_k(3*i+1:3*i+3)'/epsilon_k(i+1));
	AAA=(m_k(3,3)*m_k(1,2)^2 - 2*m_k(1,2)*m_k(1,3)*m_k(2,3) + m_k(2,2)*m_k(1,3)^2 + m_k(1,1)*m_k(2,3)^2 - m_k(1,1)*m_k(2,2)*m_k(3,3));
    r_ddot(3*i-2:3*i,1)	=   [ -(- m_k(2,3)^2 + m_k(2,2)*m_k(3,3))/AAA,    (m_k(1,2)*m_k(3,3) - m_k(1,3)*m_k(2,3))/AAA,   -(m_k(1,2)*m_k(2,3) - m_k(1,3)*m_k(2,2))/AAA;
        (m_k(1,2)*m_k(3,3) - m_k(1,3)*m_k(2,3))/AAA, -(- m_k(1,3)^2 + m_k(1,1)*m_k(3,3))/AAA,   -(m_k(1,2)*m_k(1,3) - m_k(1,1)*m_k(2,3))/AAA;
        -(m_k(1,2)*m_k(2,3) - m_k(1,3)*m_k(2,2))/AAA,   -(m_k(1,2)*m_k(1,3) - m_k(1,1)*m_k(2,3))/AAA, -(- m_k(1,2)^2 + m_k(1,1)*m_k(2,2))/AAA]*f_tol(3*i-2:3*i);
end


%% Mass matrix & acceleration
% for i = 1:numNode-1
%     m_k     =   (rho0*l(i)+0.5*C1*(epsilon_k(i)+epsilon_k(i+1)))*eye(3)-0.5*C1*(l_k(3*i-2:3*i)*l_k(3*i-2:3*i)'/epsilon_k(i)+l_k(3*i+1:3*i+3)*l_k(3*i+1:3*i+3)'/epsilon_k(i+1));
% %   (1)     r_ddot(3*i-2:3*i,1)	=	m_k\f_tol(3*i-2:3*i);
% %   (2)     
% AAA=(m_k(3,3)*m_k(1,2)^2 - 2*m_k(1,2)*m_k(1,3)*m_k(2,3) + m_k(2,2)*m_k(1,3)^2 + m_k(1,1)*m_k(2,3)^2 - m_k(1,1)*m_k(2,2)*m_k(3,3));
% r_ddot(3*i-2:3*i,1)	=   [ -(- m_k(2,3)^2 + m_k(2,2)*m_k(3,3))/AAA,    (m_k(1,2)*m_k(3,3) - m_k(1,3)*m_k(2,3))/AAA,   -(m_k(1,2)*m_k(2,3) - m_k(1,3)*m_k(2,2))/AAA;
%     (m_k(1,2)*m_k(3,3) - m_k(1,3)*m_k(2,3))/AAA, -(- m_k(1,3)^2 + m_k(1,1)*m_k(3,3))/AAA,   -(m_k(1,2)*m_k(1,3) - m_k(1,1)*m_k(2,3))/AAA;
%     -(m_k(1,2)*m_k(2,3) - m_k(1,3)*m_k(2,2))/AAA,   -(m_k(1,2)*m_k(1,3) - m_k(1,1)*m_k(2,3))/AAA, -(- m_k(1,2)^2 + m_k(1,1)*m_k(2,2))/AAA]*f_tol(3*i-2:3*i);
% 
% %   (3)
% % m1=[m_k(1,1),m_k(1,2),m_k(1,3),m_k(2,2),m_k(2,3),m_k(3,3)];F=f_tol(3*i-2:3*i);
% % a12=m_k(1,2);a13=m_k(1,3);a23=m_k(2,3);
% % m1(2)=m1(2)/m1(1);
% % m1(3)=m1(3)/m1(1);
% % F(1)=F(1)/m1(1);
% % m1(5)=(m1(5)-a12*m1(3))/(m1(4)-a12*m1(2));
% % F(2)=(F(2)-a12*F(1))/(m1(4)-a12*m1(2));		
% % m1(6)=m1(6)-a13*m1(3)-m1(5)*(a23-a13*m1(2));
% % r_ddot(3*i,1)=(F(3)-a13*F(1)-F(2)*(a23-a13*m1(2)))/m1(6);
% % r_ddot(3*i-1,1)=F(2)-m1(5)*F(3);
% % r_ddot(3*i-2,1)=F(1)-m1(2)*F(2)+m1(3)*F(3);    
% end

state_dot = [r_dot;r_ddot];

%% Seafloor resample for each node (if the seafloor is not flat)
% numNodeSeaFloor     =
% xNodeSeaFloor	=   zeros(numNodeSeaFloor,1);
% yNodeSeaFloor	=   zeros(numNodeSeaFloor,1);
% zNodeSeaFloorZ	=   zeros(numNodeSeaFloor,1);
% 
% for i=1:numNodeSeaFloor
%     xNodeSeaFloor(i,1)	=	r(3*i-2,1);
%     yNodeSeaFloor(i,1)	=   r(3*i-2,1);
% end
% zNodeSeaFloorZ  =   interp2(seaFloor(:,1),seaFloor(:,2),seaFloor(:,3),xNodeSeaFloor,yNodeSeaFloor);
% zNodeSeaFloorZ   =   waterDepth*ones(numNode+1,1);

%% Restoring forces at the top end and bottom end
% Bottom end
% Fbottom         =   E*A0*emfact*(1/l(1)-1/epsilon_k(1)) * l_k(1:3);

% Top end
Ftop            =   -E*A0*emfact*(1/l(numNode)-1/epsilon_k(numNode)) * l_k(3*numNode-2:3*numNode);
